simulink subsystem "PWM_Shifter"  (R2024b)
settings: Solver=VariableStepAuto  StartTime=0.0  StopTime=10.0  RelTol=1e-3
undefined symbols (not defined in the file or in its folder): T_pwm
libraries: simulink x3
settings Model: Creator=eric  LastModifiedBy=eric

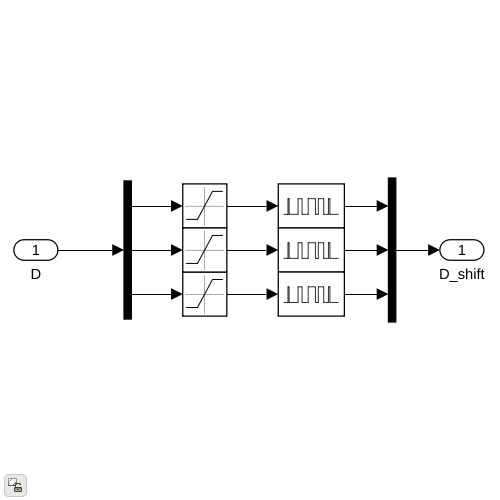
[thumbnail: Simulink's stored preview of the top-level diagram]
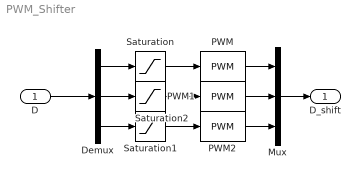
== system PWM_Shifter ==
  D : Inport
  Demux : Demux  Outputs=3
  Mux : Mux  Inputs=3
  PWM : simulink/Discontinuities/PWM  DisableCoverage=on  Period=T_pwm  InitialDelay=0  DisallowZeroDutyCycle=off  RunAtFixedTimeIntervals=off  SampleTime=T_pwm/1000
  PWM1 : simulink/Discontinuities/PWM  DisableCoverage=on  Period=T_pwm  InitialDelay=T_pwm*1/3  DisallowZeroDutyCycle=off  RunAtFixedTimeIntervals=off  SampleTime=T_pwm/1000
  PWM2 : simulink/Discontinuities/PWM  DisableCoverage=on  Period=T_pwm  InitialDelay=T_pwm*2/3  DisallowZeroDutyCycle=off  RunAtFixedTimeIntervals=off  SampleTime=T_pwm/1000
  Saturation : Saturate  UpperLimit=1  LowerLimit=0  ZeroCross=off
  Saturation1 : Saturate  UpperLimit=1  LowerLimit=0  ZeroCross=off
  Saturation2 : Saturate  UpperLimit=1  LowerLimit=0  ZeroCross=off
  D_shift : Outport
  wires:
  PWM1/1 -> Mux/2
  Demux/2 -> Saturation2/1
  Demux/3 -> Saturation1/1
  PWM/1 -> Mux/1
  PWM2/1 -> Mux/3
  Demux/1 -> Saturation/1
  D/1 -> Demux/1
  Mux/1 -> D_shift/1
  Saturation/1 -> PWM/1
  Saturation1/1 -> PWM2/1
  Saturation2/1 -> PWM1/1
